simulink model "bd_par_auto2"  (Simulink 4.1.1)
settings: Solver=ode1  SolverMode=SingleTasking  StartTime=0.0  StopTime=max(cyc_mph(:,1))  FixedStep=1  MaxStep=1  RelTol=1e-3  AbsTol=1e-3
undefined symbols (not defined in the file): air_cp, amb_tmp, cs_charge_deplete_bool, cs_charge_trq, cs_electric_decel_spd, cs_electric_launch_spd_hi, cs_electric_launch_spd_lo, cs_hi_soc, cs_lo_soc, cs_min_trq_frac, cs_off_trq_frac, cyc_avg_time, cyc_cargo_mass, cyc_elevation_init, cyc_filter_bool, cyc_grade, cyc_mph, enable_stop, ess_cap_scale, ess_coulombic_eff, ess_init_soc, ess_max_ah_cap, ess_max_volts, ess_min_volts, ess_mod_airflow, ess_mod_cp, ess_mod_init_tmp, ess_module_mass, ess_module_num, ess_on, ess_res_scale_coef, ess_res_scale_fun, ess_set_tmp, ess_th_calc, ess_th_res_off, ess_th_res_on, ess_tmp, ess_voc, ex_calc, fc_ct_trq, fc_emis, fc_inertia, fc_map_spd, fc_max_trq, fc_on, fc_spd_scale, fc_trq_scale, fc_tstat, fd_inertia, fd_loss, fd_ratio, gb_dnshift_load, gb_dnshift_spd, gb_gears_num, gb_inertia, gb_num_init, gb_ratio, gb_shift_delay, gb_spd_scale, gb_trq_scale ... (+56)
libraries: lib_wheel2 x12, lib_accessory2 x3, lib_etc x2, lib_drive_cycle2 x1, lib_interactive x1, lib_drive_cycle x1, lib_exhaust x1, lib_fuel_converter3 x1
(part 13 of 18)

== system bd_par_auto2/gearbox <gb> old/gearbox model & interface/gearbox model/gearbox controller interface ==
  T_gb_out : Inport  Port=1  LatchInput=off
  w_gb_out : Inport  Port=2  LatchInput=off
  eta_gb : Inport  Port=3  LatchInput=off
  enhancedToWorkspace1 : Subsystem  mask(enhancedToWorkspace){generalName=generalName, specificName=gear_ratio, logFlag=logFlag}
      mask prompts: generalName "General Name [char-evaluated]"; specificName "Specific Name [char-literal]"; logFlag "Enable flag (1=on,0=off)"
      mask help: A wrapper for the Simulink "To Workspace" block that allows you to evaluate the name of the variable to log to workspace. This is useful to avoid the double logging errors that occur when you pull in two library models that attempt to log to the same variable.
      mask init:
      | enhancedToWsMaker
      settings: CopyFcn=breakLinkCopyFcn  ParentCloseFcn=breakLinkParCloseFcn  RTWFcnNameOpts=Auto  RTWFileNameOpts=Auto
      mask Help:
      | <h2>Enhanced To Workspace Block</h2>
      | <h3>Parameters</h3>
      | <UL>
      | <li><b>General Name:</b> This is the more general name of the variable. Variables are saved to the workspace as <i>generalName_specificName</i>. Note that this is an evaluated variable. If you would like to type in the value directly, it must be surrounded with single quotes. Otherwise you can input the name of a variable containing a char string.</li>
      | <li><b>Specific Name:</b> This is the specific name of the variable. Note that this is input as a char literal (i.e., you don't need quotes).</li>
      | <li><b>Enable Flag:</b> This flag should have the value of 0 or 1. If 0, the variable will not be logged to the workspace. If 1, the variable will be logged. This is done so that variable logging can be turned off to improve speed.</li>
      | </ul>
      | <h3>Overview</h3>
      | <p>The enhanced to workspace block was put together to allow one to dynamically resolve variable names at run time in simulink. This is most powerful when used in conjunction with a masked subsystem to allow multiple instances of that masked subsytem to be used in the same model. The strategy is to set the generalName in the block mask which will allow the block to change the general name for all variable logging on the fly.
      | <h3>Helper Files</h3>
      | <p>Three m-files are required by the enhancedToWorkspace block. These files are located in the &lt; ADVISOR root &gt;/GUI directory :
      | <ul>
      | <li><i>enhancedToWsMaker.m</i> This file runs the mask initialization for the block</li>
      | <li><i>breakLinkCopyFcn.m</i> This file is used by the block callback when the simulink block is copied. It is necessary to break the link to the enhancedToWorkspace similar to the To Workspace block in order for it to be able to configure itself. (Try copying simulink's To Workspace block--it is impossible to make a link)</li>
      | <li><i>breakLinkParCloseFcn.m</i> This file is similar to the breakLinkCopyFcn and is used when a parent system is closed</li>
      | </ul>
      | <hr>
      | 
      | <p>Created 2003-Jan-21, Michael Patrick O'Keefe, NREL</p>
      mask Display: disp([generalName,'_',specificName])
  enhancedToWorkspace8 : Subsystem  mask(enhancedToWorkspace){generalName=generalName, specificName=shifting, logFlag=logFlag}
      mask prompts: generalName "General Name [char-evaluated]"; specificName "Specific Name [char-literal]"; logFlag "Enable flag (1=on,0=off)"
      mask help: A wrapper for the Simulink "To Workspace" block that allows you to evaluate the name of the variable to log to workspace. This is useful to avoid the double logging errors that occur when you pull in two library models that attempt to log to the same variable.
      mask init:
      | enhancedToWsMaker
      settings: CopyFcn=breakLinkCopyFcn  ParentCloseFcn=breakLinkParCloseFcn  RTWFcnNameOpts=Auto  RTWFileNameOpts=Auto
      mask Help:
      | <h2>Enhanced To Workspace Block</h2>
      | <h3>Parameters</h3>
      | <UL>
      | <li><b>General Name:</b> This is the more general name of the variable. Variables are saved to the workspace as <i>generalName_specificName</i>. Note that this is an evaluated variable. If you would like to type in the value directly, it must be surrounded with single quotes. Otherwise you can input the name of a variable containing a char string.</li>
      | <li><b>Specific Name:</b> This is the specific name of the variable. Note that this is input as a char literal (i.e., you don't need quotes).</li>
      | <li><b>Enable Flag:</b> This flag should have the value of 0 or 1. If 0, the variable will not be logged to the workspace. If 1, the variable will be logged. This is done so that variable logging can be turned off to improve speed.</li>
      | </ul>
      | <h3>Overview</h3>
      | <p>The enhanced to workspace block was put together to allow one to dynamically resolve variable names at run time in simulink. This is most powerful when used in conjunction with a masked subsystem to allow multiple instances of that masked subsytem to be used in the same model. The strategy is to set the generalName in the block mask which will allow the block to change the general name for all variable logging on the fly.
      | <h3>Helper Files</h3>
      | <p>Three m-files are required by the enhancedToWorkspace block. These files are located in the &lt; ADVISOR root &gt;/GUI directory :
      | <ul>
      | <li><i>enhancedToWsMaker.m</i> This file runs the mask initialization for the block</li>
      | <li><i>breakLinkCopyFcn.m</i> This file is used by the block callback when the simulink block is copied. It is necessary to break the link to the enhancedToWorkspace similar to the To Workspace block in order for it to be able to configure itself. (Try copying simulink's To Workspace block--it is impossible to make a link)</li>
      | <li><i>breakLinkParCloseFcn.m</i> This file is similar to the breakLinkCopyFcn and is used when a parent system is closed</li>
      | </ul>
      | <hr>
      | 
      | <p>Created 2003-Jan-21, Michael Patrick O'Keefe, NREL</p>
      mask Display: disp([generalName,'_',specificName])
  gear_ratio : Outport  Port=1  InitialOutput=0
  shifting : Outport  Port=2  InitialOutput=0
  tag scope: T_gb_out=scoped, eta_gb=scoped, w_gb_out=scoped
  wires:
  [shifting] -> enhancedToWorkspace8/1(In1), shifting/1
  T_gb_out/1 -> [T_gb_out]
  w_gb_out/1 -> [w_gb_out]
  eta_gb/1 -> [eta_gb]
  [gear_ratio] -> enhancedToWorkspace1/1(In1), gear_ratio/1

== system bd_par_auto2/gearbox <gb> old/gearbox model & interface/gearbox model/gearing (Nm) (rad/s) ==
  "output shaft torque and speed  (Nm), (rad/s)" : Inport  Port=1  LatchInput=off
  gear ratio : Inport  Port=2  LatchInput=off
  Demux : Demux  Outputs=2  BusSelectionMode=off
  Fcn1 : Fcn  Expr=1/u
  Product2 : Product  Inputs=2  Multiplication=Element-wise(.*)  SaturateOnIntegerOverflow=on
  Product3 : Product  Inputs=2  Multiplication=Element-wise(.*)  SaturateOnIntegerOverflow=on
  input shaft torque (Nm) : Outport  Port=1  InitialOutput=0
  input shaft speed (rad/s) : Outport  Port=2  InitialOutput=0
  wires:
  Demux/2 -> Product3/1
  Demux/1 -> Product2/1
  gear ratio/1 -> Product3/2, Fcn1/1
  "output shaft torque and speed  (Nm), (rad/s)"/1 -> Demux/1
  Fcn1/1 -> Product2/2
  Product2/1 -> input shaft torque (Nm)/1
  Product3/1 -> input shaft speed (rad/s)/1

== system bd_par_auto2/gearbox <gb> old/gearbox model & interface/gearbox model/gearing (Nm) (rad/s)1 ==
  input shaft torque (Nm) : Inport  Port=1  LatchInput=off
  input shaft speed (rad/s) : Inport  Port=2  LatchInput=off
  gear ratio : Inport  Port=3  LatchInput=off
  Fcn1 : Fcn  Expr=1/u
  Product2 : Product  Inputs=2  Multiplication=Element-wise(.*)  SaturateOnIntegerOverflow=on
  Product3 : Product  Inputs=2  Multiplication=Element-wise(.*)  SaturateOnIntegerOverflow=on
  output shaft torque (Nm) : Outport  Port=1  InitialOutput=0
  output shaft speed (rad/s) : Outport  Port=2  InitialOutput=0
  wires:
  input shaft speed (rad/s)/1 -> Product3/2
  input shaft torque (Nm)/1 -> Product2/1
  Product2/1 -> output shaft torque (Nm)/1
  Product3/1 -> output shaft speed (rad/s)/1
  gear ratio/1 -> Fcn1/1, Product2/2
  Fcn1/1 -> Product3/1

== system bd_par_auto2/gearbox <gb> old/gearbox model & interface/gearbox model/help ==

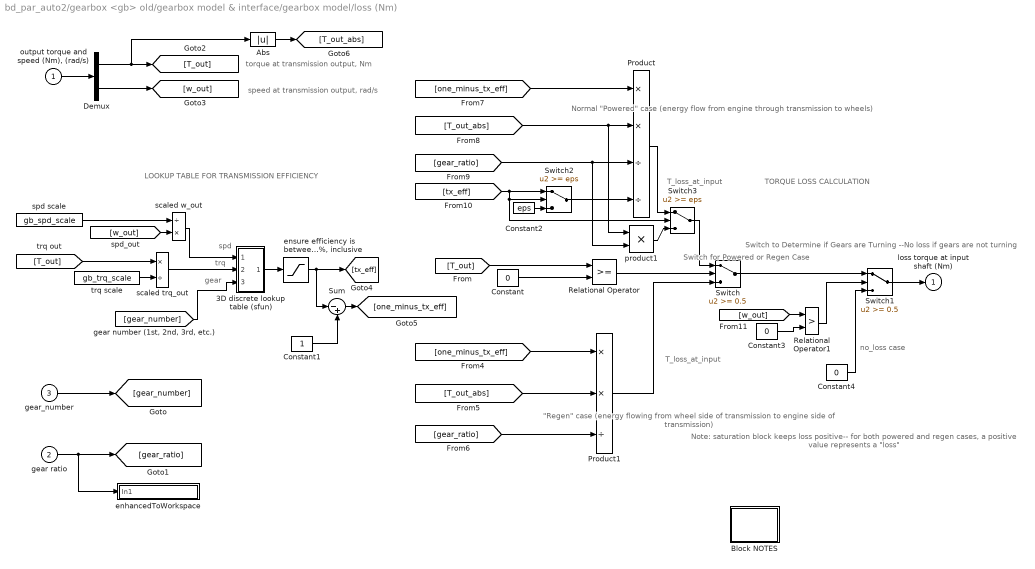
== system bd_par_auto2/gearbox <gb> old/gearbox model & interface/gearbox model/loss (Nm) ==
  note: LOOKUP TABLE FOR TRANSMISSION EFFICIENCY
  note: T_loss_at_input
  note: "Regen" case
      | (energy flowing from
      | wheel side of transmission
      | to engine side of transmission)
  note: T_loss_at_input
  note: Normal "Powered" case
      | (energy flow from engine
      | through transmission to wheels)
  note: Switch to Determine
      | if Gears are Turning
      | --No loss if gears
      | are not turning
  note: Switch for Powered
      |  or Regen Case
  note: Note: saturation block keeps
      | loss positive-- for both powered
      | and regen cases, a
      | positive value represents a "loss"
  note: no_loss case
  note: speed at transmission output, rad/s
  note: torque at transmission output, Nm
  note: spd
  note: trq
  note: gear
  note: TORQUE LOSS CALCULATION
  "output torque and speed (Nm), (rad/s)" : Inport  Port=1  LatchInput=off
  gear ratio : Inport  Port=2  LatchInput=off
  gear_number : Inport  Port=3  LatchInput=off
  3D discrete lookup table (sfun) : Subsystem  mask{tx_map_spd=tx_map_spd, tx_map_trq=tx_map_trq, tx_eff_map=tx_eff_map}
      mask prompts: tx_map_spd "Row Lookup"; tx_map_trq "Column Lookup"; tx_eff_map "Lookup Matrix"
      settings: RTWFcnNameOpts=Auto  RTWFileNameOpts=Auto
  Abs : Abs  SaturateOnIntegerOverflow=on
  Block NOTES : Subsystem
      settings: RTWFcnNameOpts=Auto  RTWFileNameOpts=Auto
      mask Display: disp('Block\nNOTES')
  Constant : Constant  Value=0
  Constant1 : Constant  Value=1
  Constant2 : Constant  Value=eps
  Constant3 : Constant  Value=0
  Constant4 : Constant  Value=0
  Demux : Demux  Outputs=2  BusSelectionMode=off
  Product : Product  Inputs=**//  Multiplication=Element-wise(.*)  SaturateOnIntegerOverflow=on
  Product1 : Product  Inputs=**/  Multiplication=Element-wise(.*)  SaturateOnIntegerOverflow=on
  Relational Operator : RelationalOperator  Operator=>=
  Relational Operator1 : RelationalOperator  Operator=>
  Sum : Sum  Inputs=|-+  SaturateOnIntegerOverflow=on
  Switch : Switch  Threshold=0.5
  Switch1 : Switch  Threshold=0.5
  Switch2 : Switch  Threshold=eps
  Switch3 : Switch  Threshold=eps
  enhancedToWorkspace : Subsystem  TreatAsAtomicUnit=on  mask(enhancedToWorkspace){generalName=generalName, specificName=current_gear_ratio, logFlag=logFlag}
      mask prompts: generalName "General Name [char-evaluated]"; specificName "Specific Name [char-literal]"; logFlag "Enable flag (1=on,0=off)"
      mask help: A wrapper for the Simulink "To Workspace" block that allows you to evaluate the name of the variable to log to workspace. This is useful to avoid the double logging errors that occur when you pull in two library models that attempt to log to the same variable.
      mask init:
      | enhancedToWsMaker
      settings: CopyFcn=breakLinkCopyFcn  ParentCloseFcn=breakLinkParCloseFcn  RTWFcnNameOpts=Auto  RTWFileNameOpts=Auto
      mask Help:
      | <h2>Enhanced To Workspace Block</h2>
      | <h3>Parameters</h3>
      | <UL>
      | <li><b>General Name:</b> This is the more general name of the variable. Variables are saved to the workspace as <i>generalName_specificName</i>. Note that this is an evaluated variable. If you would like to type in the value directly, it must be surrounded with single quotes. Otherwise you can input the name of a variable containing a char string.</li>
      | <li><b>Specific Name:</b> This is the specific name of the variable. Note that this is input as a char literal (i.e., you don't need quotes).</li>
      | <li><b>Enable Flag:</b> This flag should have the value of 0 or 1. If 0, the variable will not be logged to the workspace. If 1, the variable will be logged. This is done so that variable logging can be turned off to improve speed.</li>
      | </ul>
      | <h3>Overview</h3>
      | <p>The enhanced to workspace block was put together to allow one to dynamically resolve variable names at run time in simulink. This is most powerful when used in conjunction with a masked subsystem to allow multiple instances of that masked subsytem to be used in the same model. The strategy is to set the generalName in the block mask which will allow the block to change the general name for all variable logging on the fly.
      | <h3>Helper Files</h3>
      | <p>Three m-files are required by the enhancedToWorkspace block. These files are located in the &lt; ADVISOR root &gt;/GUI directory :
      | <ul>
      | <li><i>enhancedToWsMaker.m</i> This file runs the mask initialization for the block</li>
      | <li><i>breakLinkCopyFcn.m</i> This file is used by the block callback when the simulink block is copied. It is necessary to break the link to the enhancedToWorkspace similar to the To Workspace block in order for it to be able to configure itself. (Try copying simulink's To Workspace block--it is impossible to make a link)</li>
      | <li><i>breakLinkParCloseFcn.m</i> This file is similar to the breakLinkCopyFcn and is used when a parent system is closed</li>
      | </ul>
      | <hr>
      | 
      | <p>Created 2003-Jan-21, Michael Patrick O'Keefe, NREL</p>
      | 
      | <!--
      | <VARDEF>
      | <H3>var_name</H3>
      | <UL>
      | <LI><B>data type</B> data type here</LI>
      | <LI><B>units</B> units here</LI>
      | <LI><B>vehicle type</B> vehicle type here</LI>
      | <LI><B>description</B> description here</LI>
      | </UL>
      | </VARDEF>
      | -->
      mask Display: disp([generalName,'_',specificName])
  "ensure efficiency is between  0% and 100%, inclusive" : Saturate  UpperLimit=1  LowerLimit=0  LinearizeAsGain=on
  product1 : Product  Inputs=2  Multiplication=Element-wise(.*)  SaturateOnIntegerOverflow=on
  scaled trq_out : Product  Inputs=*/  Multiplication=Element-wise(.*)  SaturateOnIntegerOverflow=on
  scaled w_out : Product  Inputs=/*  Multiplication=Element-wise(.*)  SaturateOnIntegerOverflow=on
  spd scale : Constant  Value=gb_spd_scale
  trq scale : Constant  Value=gb_trq_scale
  loss torque at input shaft (Nm) : Outport  Port=1  InitialOutput=0
  wires:
  "output torque and speed (Nm), (rad/s)"/1 -> Demux/1
  Demux/2 -> [w_out]
  [gear_number] -> 3D discrete lookup table (sfun)/3("gear_number  (e.g., 1, 2, 3)")
  Relational Operator/1 -> Switch/2
  Constant/1 -> Relational Operator/2
  [T_out] -> Relational Operator/1
  Product1/1 -> Switch/3
  [one_minus_tx_eff] -> Product1/1
  [gear_ratio] -> Product1/3
  [T_out_abs] -> Product1/2
  [one_minus_tx_eff] -> Product/1
  [T_out_abs] -> Product/2, product1/1
  [gear_ratio] -> Product/3, product1/2
  Switch1/1 -> loss torque at input shaft (Nm)/1
  Constant4/1 -> Switch1/3
  [w_out] -> Relational Operator1/1
  Constant3/1 -> Relational Operator1/2
  Relational Operator1/1 -> Switch1/2
  Demux/1 -> [T_out], Abs/1
  Abs/1 -> [T_out_abs]
  Switch/1 -> Switch1/1
  3D discrete lookup table (sfun)/1(tx_eff) -> "ensure efficiency is between  0% and 100%, inclusive"/1
  "ensure efficiency is between  0% and 100%, inclusive"/1 -> [tx_eff], Sum/1
  scaled w_out/1 -> 3D discrete lookup table (sfun)/1(lookup speed (rad/s))
  [T_out] -> scaled trq_out/1
  scaled trq_out/1 -> 3D discrete lookup table (sfun)/2(lookup trq (Nm))
  trq scale/1 -> scaled trq_out/2
  Constant1/1 -> Sum/2
  Sum/1 -> [one_minus_tx_eff]
  [w_out] -> scaled w_out/2
  spd scale/1 -> scaled w_out/1
  gear ratio/1 -> enhancedToWorkspace/1(In1), [gear_ratio]
  gear_number/1 -> [gear_number]
  Switch2/1 -> Product/4
  [tx_eff] -> Switch2/1, Switch2/2, Switch3/2
  Constant2/1 -> Switch2/3
  Switch3/1 -> Switch/1
  Product/1 -> Switch3/1
  product1/1 -> Switch3/3

== system bd_par_auto2/hydraulic torque converter <htc> HEV/HTC for parallel HEV and Interface/model for parallel HEV/Block NOTES ==
  note: This block predicts the relative speed of the HTC input (pump) and output
      | (turbine).  Torque converter lockup is modeled.

== system bd_par_auto2/hydraulic torque converter <htc> HEV/HTC for parallel HEV and Interface/model for parallel HEV/SR ==
  T,w req out : Inport  Port=1  LatchInput=off
  w in : Inport  Port=2  LatchInput=off
  >0 : Saturate  UpperLimit=inf  LowerLimit=eps  LinearizeAsGain=on
  Constant : Constant  Orientation=left  Value=0
  Constant1 : Constant  Value=vc_idle_spd+eps
  Constant3 : Constant  Value=1
  K_adv : Subsystem
      settings: RTWFcnNameOpts=Auto  RTWFileNameOpts=Auto
  K_adv_coast : Subsystem
      settings: RTWFcnNameOpts=Auto  RTWFileNameOpts=Auto
  Logical Operator : Logic  Operator=NOT  Inputs=1
  Logical Operator1 : Logic  Operator=NOT  Inputs=1
  MinMax : MinMax  Function=min  Inputs=2
  Relational Operator : RelationalOperator  Operator=>=
  SR Look-Up Table SR=wout/win : Lookup  InputValues=htc_k_adv  OutputValues=htc_sr
  SR Look-Up Table SR=wout/win coast : Lookup  InputValues=fliplr(htc_k_adv_coast)  OutputValues=fliplr(htc_sr_coast)
  SRmax= wout/win,min : Product  Inputs=*/  Multiplication=Element-wise(.*)  SaturateOnIntegerOverflow=on
  T : Selector  InputType=Vector  ElementSrc=Internal  Elements=1  RowSrc=Internal  Rows=1  ColumnSrc=Internal  Columns=1  InputPortWidth=2
  enhancedToWorkspace : Subsystem  TreatAsAtomicUnit=on  mask(enhancedToWorkspace){generalName=generalName, specificName=locked, logFlag=logFlag}
      mask prompts: generalName "General Name [char-evaluated]"; specificName "Specific Name [char-literal]"; logFlag "Enable flag (1=on,0=off)"
      mask help: A wrapper for the Simulink "To Workspace" block that allows you to evaluate the name of the variable to log to workspace. This is useful to avoid the double logging errors that occur when you pull in two library models that attempt to log to the same variable.
      mask init:
      | enhancedToWsMaker
      settings: CopyFcn=breakLinkCopyFcn  ParentCloseFcn=breakLinkParCloseFcn  RTWFcnNameOpts=Auto  RTWFileNameOpts=Auto
      mask Help:
      | <h2>Enhanced To Workspace Block</h2>
      | <h3>Parameters</h3>
      | <UL>
      | <li><b>General Name:</b> This is the more general name of the variable. Variables are saved to the workspace as <i>generalName_specificName</i>. Note that this is an evaluated variable. If you would like to type in the value directly, it must be surrounded with single quotes. Otherwise you can input the name of a variable containing a char string.</li>
      | <li><b>Specific Name:</b> This is the specific name of the variable. Note that this is input as a char literal (i.e., you don't need quotes).</li>
      | <li><b>Enable Flag:</b> This flag should have the value of 0 or 1. If 0, the variable will not be logged to the workspace. If 1, the variable will be logged. This is done so that variable logging can be turned off to improve speed.</li>
      | </ul>
      | <h3>Overview</h3>
      | <p>The enhanced to workspace block was put together to allow one to dynamically resolve variable names at run time in simulink. This is most powerful when used in conjunction with a masked subsystem to allow multiple instances of that masked subsytem to be used in the same model. The strategy is to set the generalName in the block mask which will allow the block to change the general name for all variable logging on the fly.
      | <h3>Helper Files</h3>
      | <p>Three m-files are required by the enhancedToWorkspace block. These files are located in the &lt; ADVISOR root &gt;/GUI directory :
      | <ul>
      | <li><i>enhancedToWsMaker.m</i> This file runs the mask initialization for the block</li>
      | <li><i>breakLinkCopyFcn.m</i> This file is used by the block callback when the simulink block is copied. It is necessary to break the link to the enhancedToWorkspace similar to the To Workspace block in order for it to be able to configure itself. (Try copying simulink's To Workspace block--it is impossible to make a link)</li>
      | <li><i>breakLinkParCloseFcn.m</i> This file is similar to the breakLinkCopyFcn and is used when a parent system is closed</li>
      | </ul>
      | <hr>
      | 
      | <p>Created 2003-Jan-21, Michael Patrick O'Keefe, NREL</p>
      | 
      | <!--
      | <VARDEF>
      | <H3>var_name</H3>
      | <UL>
      | <LI><B>data type</B> data type here</LI>
      | <LI><B>units</B> units here</LI>
      | <LI><B>vehicle type</B> vehicle type here</LI>
      | <LI><B>description</B> description here</LI>
      | </UL>
      | </VARDEF>
      | -->
      mask Display: disp([generalName,'_',specificName])
  enhancedToWorkspace1 : Subsystem  TreatAsAtomicUnit=on  mask(enhancedToWorkspace){generalName=generalName, specificName=coasting, logFlag=logFlag}
      mask prompts: generalName "General Name [char-evaluated]"; specificName "Specific Name [char-literal]"; logFlag "Enable flag (1=on,0=off)"
      mask help: A wrapper for the Simulink "To Workspace" block that allows you to evaluate the name of the variable to log to workspace. This is useful to avoid the double logging errors that occur when you pull in two library models that attempt to log to the same variable.
      mask init:
      | enhancedToWsMaker
      settings: CopyFcn=breakLinkCopyFcn  ParentCloseFcn=breakLinkParCloseFcn  RTWFcnNameOpts=Auto  RTWFileNameOpts=Auto
      mask Help:
      | <h2>Enhanced To Workspace Block</h2>
      | <h3>Parameters</h3>
      | <UL>
      | <li><b>General Name:</b> This is the more general name of the variable. Variables are saved to the workspace as <i>generalName_specificName</i>. Note that this is an evaluated variable. If you would like to type in the value directly, it must be surrounded with single quotes. Otherwise you can input the name of a variable containing a char string.</li>
      | <li><b>Specific Name:</b> This is the specific name of the variable. Note that this is input as a char literal (i.e., you don't need quotes).</li>
      | <li><b>Enable Flag:</b> This flag should have the value of 0 or 1. If 0, the variable will not be logged to the workspace. If 1, the variable will be logged. This is done so that variable logging can be turned off to improve speed.</li>
      | </ul>
      | <h3>Overview</h3>
      | <p>The enhanced to workspace block was put together to allow one to dynamically resolve variable names at run time in simulink. This is most powerful when used in conjunction with a masked subsystem to allow multiple instances of that masked subsytem to be used in the same model. The strategy is to set the generalName in the block mask which will allow the block to change the general name for all variable logging on the fly.
      | <h3>Helper Files</h3>
      | <p>Three m-files are required by the enhancedToWorkspace block. These files are located in the &lt; ADVISOR root &gt;/GUI directory :
      | <ul>
      | <li><i>enhancedToWsMaker.m</i> This file runs the mask initialization for the block</li>
      | <li><i>breakLinkCopyFcn.m</i> This file is used by the block callback when the simulink block is copied. It is necessary to break the link to the enhancedToWorkspace similar to the To Workspace block in order for it to be able to configure itself. (Try copying simulink's To Workspace block--it is impossible to make a link)</li>
      | <li><i>breakLinkParCloseFcn.m</i> This file is similar to the breakLinkCopyFcn and is used when a parent system is closed</li>
      | </ul>
      | <hr>
      | 
      | <p>Created 2003-Jan-21, Michael Patrick O'Keefe, NREL</p>
      | 
      | <!--
      | <VARDEF>
      | <H3>var_name</H3>
      | <UL>
      | <LI><B>data type</B> data type here</LI>
      | <LI><B>units</B> units here</LI>
      | <LI><B>vehicle type</B> vehicle type here</LI>
      | <LI><B>description</B> description here</LI>
      | </UL>
      | </VARDEF>
      | -->
      mask Display: disp([generalName,'_',specificName])
  if coasting : Switch  Threshold=eps
  "locked up, then SR=1" : Switch  Threshold=eps
  min,max : Saturate  UpperLimit=inf  LowerLimit=1  LinearizeAsGain=on
  shifting SR : Subsystem
      settings: RTWFcnNameOpts=Auto  RTWFileNameOpts=Auto
  wout,req : Selector  InputType=Vector  ElementSrc=Internal  Elements=2  RowSrc=Internal  Rows=1  ColumnSrc=Internal  Columns=1  InputPortWidth=2
  SR : Outport  Port=1  InitialOutput=0
  coasting : Outport  Port=2  InitialOutput=0
  wires:
  Relational Operator/1 -> if coasting/2, Logical Operator1/1
  [locked_up] -> enhancedToWorkspace/1(In1), Logical Operator/1
  T,w req out/1 -> T/1, K_adv_coast/1("Req'd output trq and spd (Nm), (rad/s)"), wout,req/1, K_adv/1("Req'd output trq and spd (Nm), (rad/s)"), shifting SR/1(T,w req out)
  SR Look-Up Table SR=wout/win coast/1 -> min,max/1
  Constant/1 -> Relational Operator/2
  T/1 -> Relational Operator/1
  Logical Operator/1 -> "locked up, then SR=1"/2
  Constant3/1 -> "locked up, then SR=1"/3
  SR Look-Up Table SR=wout/win/1 -> "locked up, then SR=1"/1
  w in/1 -> shifting SR/2(w in)
  "locked up, then SR=1"/1 -> shifting SR/3(SR)
  shifting SR/1(SR limited) -> if coasting/1
  SRmax= wout/win,min/1 -> MinMax/2
  Constant1/1 -> SRmax= wout/win,min/2
  wout,req/1 -> SRmax= wout/win,min/1
  min,max/1 -> MinMax/1
  MinMax/1 -> if coasting/3
  K_adv_coast/1(K_adv_coast) -> SR Look-Up Table SR=wout/win coast/1
  if coasting/1 -> >0/1
  >0/1 -> SR/1
  Logical Operator1/1 -> enhancedToWorkspace1/1(In1), coasting/1
  K_adv/1(K_adv) -> SR Look-Up Table SR=wout/win/1

== system bd_par_auto2/hydraulic torque converter <htc> HEV/HTC for parallel HEV and Interface/model for parallel HEV/T, shifting ==
  TR : Inport  Port=1  LatchInput=off
  Req'd  input trq : Inport  Port=2  LatchInput=off
  Req'd output trq : Inport  Port=3  LatchInput=off
  htc_spd_in_a : Inport  Port=4  LatchInput=off
  SR : Inport  Port=5  LatchInput=off
  Memory : Memory  X0=0  InheritSampleTime=off
      settings: RTWStateStorageClass=Auto
  Memory1 : Memory  X0=0  InheritSampleTime=off
      settings: RTWStateStorageClass=Auto
  MinMax : MinMax  Function=min  Inputs=2
  TR Look-Up Table TR=Tout/Tin : Lookup  InputValues=htc_sr  OutputValues=htc_tr
  T_max : Subsystem
      settings: RTWFcnNameOpts=Auto  RTWFileNameOpts=Auto
  Tin*TR= Tout,req : Product  Inputs=2  Multiplication=Element-wise(.*)  SaturateOnIntegerOverflow=on
  engine speed estimator : Subsystem
      settings: RTWFcnNameOpts=Auto  RTWFileNameOpts=Auto
  "shifting, override zero Trequest" : Switch  Threshold=eps
  T req : Outport  Port=1
  wires:
  [shifting] -> "shifting, override zero Trequest"/2
  Req'd output trq/1 -> "shifting, override zero Trequest"/3
  htc_spd_in_a/1 -> engine speed estimator/1(htc_spd_in_a)
  SR/1 -> Memory1/1
  Memory1/1 -> TR Look-Up Table TR=Tout/Tin/1
  engine speed estimator/1(Out1) -> T_max/1(w_APU)
  MinMax/1 -> T req/1
  TR Look-Up Table TR=Tout/Tin/1 -> T_max/2(TR)
  "shifting, override zero Trequest"/1 -> MinMax/1
  T_max/1(T_max max gain from htc) -> MinMax/2
  Memory/1 -> "shifting, override zero Trequest"/1
  Req'd  input trq/1 -> Tin*TR= Tout,req/1
  TR/1 -> Tin*TR= Tout,req/2
  Tin*TR= Tout,req/1 -> Memory/1

== system bd_par_auto2/hydraulic torque converter <htc> HEV/HTC for parallel HEV and Interface/model for parallel HEV/TR ==
  SR : Inport  Port=1  LatchInput=off
  coasting : Inport  Port=2  LatchInput=off
  1/SR*TR  for coast : Fcn  Expr=1/u
  Constant3 : Constant  Value=1
  Logical Operator : Logic  Operator=NOT  Inputs=1
  Logical Operator1 : Logic  Operator=NOT  Inputs=1
  TR Look-Up Table TR=Tout/Tin : Lookup  InputValues=htc_sr  OutputValues=htc_tr
  TR Look-Up Table TR=Tout/Tin coast : Lookup  InputValues=htc_sr_coast  OutputValues=htc_tr_coast
  To Workspace11 : ToWorkspace  VariableName=htc_efficiency  SampleTime=-1  SaveFormat=Array
  effic=SR*TR : Product  Inputs=**  Multiplication=Element-wise(.*)  SaturateOnIntegerOverflow=on
  if coasting : Switch  Threshold=eps
  if coasting1 : Switch  Threshold=eps
  "locked up, then TR=1" : Switch  Threshold=eps
  min,max : Saturate  UpperLimit=htc_max_coast_tr  LowerLimit=htc_min_coast_tr  LinearizeAsGain=on
  TR : Outport  Port=1  InitialOutput=0
  wires:
  TR Look-Up Table TR=Tout/Tin/1 -> "locked up, then TR=1"/1
  Constant3/1 -> "locked up, then TR=1"/3
  [locked_up] -> Logical Operator/1
  Logical Operator/1 -> "locked up, then TR=1"/2
  "locked up, then TR=1"/1 -> if coasting/1
  TR Look-Up Table TR=Tout/Tin coast/1 -> min,max/1
  min,max/1 -> if coasting/3
  SR/1 -> TR Look-Up Table TR=Tout/Tin coast/1, TR Look-Up Table TR=Tout/Tin/1, effic=SR*TR/1
  coasting/1 -> Logical Operator1/1
  if coasting/1 -> TR/1, effic=SR*TR/2
  Logical Operator1/1 -> if coasting/2, if coasting1/2
  effic=SR*TR/1 -> if coasting1/1, 1/SR*TR  for coast/1
  1/SR*TR  for coast/1 -> if coasting1/3
  if coasting1/1 -> To Workspace11/1

== system bd_par_auto2/hydraulic torque converter <htc> HEV/HTC for parallel HEV and Interface/model for parallel HEV/effect of inertia (Nm) ==
  note: This block computes the torque required to overcome the inertia of the
      | turbine (plus 1/2 fluid in htc).
  turbine/output speed (rad/s) : Inport  Port=1  LatchInput=off
  Constant : Constant  Value=htc_inertia
  Product : Product  Inputs=2  Multiplication=Element-wise(.*)  SaturateOnIntegerOverflow=on
  d/dt : Derivative
  inertia torque (Nm) : Outport  Port=1  InitialOutput=0
  wires:
  d/dt/1 -> Product/1
  turbine/output speed (rad/s)/1 -> d/dt/1
  Constant/1 -> Product/2
  Product/1 -> inertia torque (Nm)/1

== system bd_par_auto2/hydraulic torque converter <htc> HEV/HTC for parallel HEV and Interface/model for parallel HEV/enhancedToWorkspace ==
  In1 : Inport  Port=1  LatchInput=off
  To Workspace : ToWorkspace  VariableName=htc_spd_in_a  SampleTime=-1  SaveFormat=Array
  wires:
  In1/1 -> To Workspace/1

== system bd_par_auto2/hydraulic torque converter <htc> HEV/HTC for parallel HEV and Interface/model for parallel HEV/enhancedToWorkspace1 ==
  In1 : Inport  Port=1  LatchInput=off
  To Workspace : ToWorkspace  VariableName=htc_trq_in_a  SampleTime=-1  SaveFormat=Array
  wires:
  In1/1 -> To Workspace/1

== system bd_par_auto2/hydraulic torque converter <htc> HEV/HTC for parallel HEV and Interface/model for parallel HEV/enhancedToWorkspace10 ==
  In1 : Inport  Port=1  LatchInput=off
  To Workspace : ToWorkspace  VariableName=htc_trq_in_r  SampleTime=-1  SaveFormat=Array
  wires:
  In1/1 -> To Workspace/1

== system bd_par_auto2/hydraulic torque converter <htc> HEV/HTC for parallel HEV and Interface/model for parallel HEV/enhancedToWorkspace2 ==
  In1 : Inport  Port=1  LatchInput=off
  To Workspace : ToWorkspace  VariableName=htc_sr_hist  SampleTime=-1  SaveFormat=Array
  wires:
  In1/1 -> To Workspace/1

== system bd_par_auto2/hydraulic torque converter <htc> HEV/HTC for parallel HEV and Interface/model for parallel HEV/enhancedToWorkspace3 ==
  In1 : Inport  Port=1  LatchInput=off
  To Workspace : ToWorkspace  VariableName=htc_tr_hist  SampleTime=-1  SaveFormat=Array
  wires:
  In1/1 -> To Workspace/1

== system bd_par_auto2/hydraulic torque converter <htc> HEV/HTC for parallel HEV and Interface/model for parallel HEV/enhancedToWorkspace4 ==
  In1 : Inport  Port=1  LatchInput=off
  To Workspace : ToWorkspace  VariableName=htc_trq_inertia  SampleTime=-1  SaveFormat=Array
  wires:
  In1/1 -> To Workspace/1

== system bd_par_auto2/hydraulic torque converter <htc> HEV/HTC for parallel HEV and Interface/model for parallel HEV/enhancedToWorkspace5 ==
  In1 : Inport  Port=1  LatchInput=off
  To Workspace : ToWorkspace  VariableName=htc_trq_out_a  SampleTime=-1  SaveFormat=Array
  wires:
  In1/1 -> To Workspace/1

== system bd_par_auto2/hydraulic torque converter <htc> HEV/HTC for parallel HEV and Interface/model for parallel HEV/enhancedToWorkspace6 ==
  In1 : Inport  Port=1  LatchInput=off
  To Workspace : ToWorkspace  VariableName=htc_spd_out_a  SampleTime=-1  SaveFormat=Array
  wires:
  In1/1 -> To Workspace/1

== system bd_par_auto2/hydraulic torque converter <htc> HEV/HTC for parallel HEV and Interface/model for parallel HEV/enhancedToWorkspace7 ==
  In1 : Inport  Port=1  LatchInput=off
  To Workspace : ToWorkspace  VariableName=htc_trq_out_r  SampleTime=-1  SaveFormat=Array
  wires:
  In1/1 -> To Workspace/1

== system bd_par_auto2/hydraulic torque converter <htc> HEV/HTC for parallel HEV and Interface/model for parallel HEV/enhancedToWorkspace8 ==
  In1 : Inport  Port=1  LatchInput=off
  To Workspace : ToWorkspace  VariableName=htc_spd_out_r  SampleTime=-1  SaveFormat=Array
  wires:
  In1/1 -> To Workspace/1

== system bd_par_auto2/hydraulic torque converter <htc> HEV/HTC for parallel HEV and Interface/model for parallel HEV/enhancedToWorkspace9 ==
  In1 : Inport  Port=1  LatchInput=off
  To Workspace : ToWorkspace  VariableName=htc_spd_in_r  SampleTime=-1  SaveFormat=Array
  wires:
  In1/1 -> To Workspace/1

== system bd_par_auto2/motor/controller <mc>/motor model & interface/mc model/Block NOTES ==
  note: Available torque is computed from available power by assuming that the ratio of rotor torque to input
      | (electric) power is the same for the actual/achievable situation as was computed for the request.  This
      | is mathematically equivalent to assuming that the motor/controller efficiency.  Rotor speed for the
      | actual/achievable calculations is as computed in the 'request' branch.
  note: This motor/controller model includes loss data, rotational inertia, and performance limits.

== system bd_par_auto2/motor/controller <mc>/motor model & interface/mc model/N-m drive torque per W input ==
  req'd input power (W) : Inport  Port=1  LatchInput=off
  req'd rotor drive torque (Nm) : Inport  Port=2  LatchInput=off
  Block NOTES : Subsystem
      settings: RTWFcnNameOpts=Auto  RTWFileNameOpts=Auto
      mask Display: disp('Block\nNOTES')
  Constant : Constant  Value=eps
  Constant1 : Constant  Value=0
  Constant2 : Constant  Value=inf
  Product : Product  Inputs=/*  Multiplication=Element-wise(.*)  SaturateOnIntegerOverflow=on
  Relational Operator : RelationalOperator  Operator=~=
  Sum : Sum  Inputs=++  SaturateOnIntegerOverflow=on
  Switch : Switch  Threshold=eps
  Nm per W : Outport  Port=1  InitialOutput=0
  wires:
  Constant2/1 -> Switch/3
  Constant1/1 -> Relational Operator/2
  req'd input power (W)/1 -> Relational Operator/1, Sum/2
  Sum/1 -> Product/1
  Switch/1 -> Nm per W/1
  Relational Operator/1 -> Switch/2
  Product/1 -> Switch/1
  req'd rotor drive torque (Nm)/1 -> Product/2
  Constant/1 -> Sum/1

== system bd_par_auto2/motor/controller <mc>/motor model & interface/mc model/documentation10 ==

== system bd_par_auto2/motor/controller <mc>/motor model & interface/mc model/effect of inertia (Nm) ==
  mc_spd_out_a : Inport  Port=1  LatchInput=off
  Block NOTES : Subsystem
      settings: RTWFcnNameOpts=Auto  RTWFileNameOpts=Auto
      mask Display: disp('Block\nNOTES')
  Constant : Constant  Value=eps
  Constant1 : Constant  Value=max(mc_max_trq)*mc_trq_scale*mc_overtrq_factor
  Constant2 : Constant  Orientation=left  Value=gb_ratio(1)*fd_ratio/wh_radius
  Gain : Gain  Gain=mc_inertia  Multiplication=Element-wise(K.*u)  SaturateOnIntegerOverflow=on
  Memory : Memory  X0=0  InheritSampleTime=off
      settings: RTWStateStorageClass=Auto
  MinMax : MinMax  Function=min  Inputs=2
  Product : Product  Inputs=2  Multiplication=Element-wise(.*)  SaturateOnIntegerOverflow=on
  Sum : Sum  Inputs=++  SaturateOnIntegerOverflow=on
  Switch : Switch  Threshold=eps
  alpha : Derivative
  motor inertia as a function of total vehicle inertia (generous approximation) : Subsystem  Orientation=up
      settings: RTWFcnNameOpts=Auto  RTWFileNameOpts=Auto
  overall gear ratio / wh_radius : Product  Inputs=*/  Multiplication=Element-wise(.*)  SaturateOnIntegerOverflow=on
  out_1 : Outport  Port=1  InitialOutput=0
  wires:
  Switch/1 -> overall gear ratio / wh_radius/2
  Constant2/1 -> Switch/3
  [veh_spd_a_rec_prev] -> Switch/2, Sum/1
  Sum/1 -> Switch/1
  Constant/1 -> Sum/2
  motor inertia as a function of total vehicle inertia (generous approximation)/1(Out1) -> Product/2
  Constant1/1 -> Product/1
  overall gear ratio / wh_radius/1 -> motor inertia as a function of total vehicle inertia (generous approximation)/1(gear ratio)
  Product/1 -> MinMax/2
  Gain/1 -> MinMax/1
  MinMax/1 -> out_1/1
  mc_spd_out_a/1 -> alpha/1, Memory/1
  alpha/1 -> Gain/1
  Memory/1 -> overall gear ratio / wh_radius/1

== system bd_par_auto2/motor/controller <mc>/motor model & interface/mc model/enforce torque limit ==
  req'd motor torque (Nm) : Inport  Port=1  LatchInput=off
  limited motor speed (rad/s) : Inport  Port=2  LatchInput=off
  Block NOTES : Subsystem
      settings: RTWFcnNameOpts=Auto  RTWFileNameOpts=Auto
      mask Display: disp('Block\nNOTES')
  MinMax : MinMax  Function=min  Inputs=2
  MinMax1 : MinMax  Function=max  Inputs=2
  Relational Operator2 : RelationalOperator  Operator=~=
  Switch : Switch  Threshold=0
  enhancedToWorkspace : Subsystem  mask(enhancedToWorkspace){generalName=generalName, specificName=max_trq_vec, logFlag=logFlag}
      mask prompts: generalName "General Name [char-evaluated]"; specificName "Specific Name [char-literal]"; logFlag "Enable flag (1=on,0=off)"
      mask help: A wrapper for the Simulink "To Workspace" block that allows you to evaluate the name of the variable to log to workspace. This is useful to avoid the double logging errors that occur when you pull in two library models that attempt to log to the same variable.
      mask init:
      | enhancedToWsMaker
      settings: CopyFcn=breakLinkCopyFcn  ParentCloseFcn=breakLinkParCloseFcn  RTWFcnNameOpts=Auto  RTWFileNameOpts=Auto
      mask Help:
      | <h2>Enhanced To Workspace Block</h2>
      | <h3>Parameters</h3>
      | <UL>
      | <li><b>General Name:</b> This is the more general name of the variable. Variables are saved to the workspace as <i>generalName_specificName</i>. Note that this is an evaluated variable. If you would like to type in the value directly, it must be surrounded with single quotes. Otherwise you can input the name of a variable containing a char string.</li>
      | <li><b>Specific Name:</b> This is the specific name of the variable. Note that this is input as a char literal (i.e., you don't need quotes).</li>
      | <li><b>Enable Flag:</b> This flag should have the value of 0 or 1. If 0, the variable will not be logged to the workspace. If 1, the variable will be logged. This is done so that variable logging can be turned off to improve speed.</li>
      | </ul>
      | <h3>Overview</h3>
      | <p>The enhanced to workspace block was put together to allow one to dynamically resolve variable names at run time in simulink. This is most powerful when used in conjunction with a masked subsystem to allow multiple instances of that masked subsytem to be used in the same model. The strategy is to set the generalName in the block mask which will allow the block to change the general name for all variable logging on the fly.
      | <h3>Helper Files</h3>
      | <p>Three m-files are required by the enhancedToWorkspace block. These files are located in the &lt; ADVISOR root &gt;/GUI directory :
      | <ul>
      | <li><i>enhancedToWsMaker.m</i> This file runs the mask initialization for the block</li>
      | <li><i>breakLinkCopyFcn.m</i> This file is used by the block callback when the simulink block is copied. It is necessary to break the link to the enhancedToWorkspace similar to the To Workspace block in order for it to be able to configure itself. (Try copying simulink's To Workspace block--it is impossible to make a link)</li>
      | <li><i>breakLinkParCloseFcn.m</i> This file is similar to the breakLinkCopyFcn and is used when a parent system is closed</li>
      | </ul>
      | <hr>
      | 
      | <p>Created 2003-Jan-21, Michael Patrick O'Keefe, NREL</p>
      mask Display: disp([generalName,'_',specificName])
  max gen torque : Lookup  InputValues=mc_map_spd*mc_spd_scale  OutputValues=mc_max_gen_trq*mc_overtrq_factor*mc_trq_scale
  max torque : Lookup  InputValues=mc_map_spd*mc_spd_scale  OutputValues=mc_max_trq*mc_overtrq_factor*mc_trq_scale
  limited motor torque (Nm) : Outport  Port=1
  tag scope: mc_trq_limited=scoped
  wires:
  max gen torque/1 -> MinMax1/2
  limited motor speed (rad/s)/1 -> max gen torque/1, max torque/1
  Relational Operator2/1 -> [mc_trq_limited]
  MinMax/1 -> Switch/1
  MinMax1/1 -> Switch/3
  Switch/1 -> limited motor torque (Nm)/1, Relational Operator2/2
  req'd motor torque (Nm)/1 -> MinMax/1, MinMax1/1, Switch/2, Relational Operator2/1
  max torque/1 -> enhancedToWorkspace/1(In1), MinMax/2

== system bd_par_auto2/motor/controller <mc>/motor model & interface/mc model/enhancedToWorkspace ==
  In1 : Inport  Port=1  LatchInput=off
  To Workspace : ToWorkspace  VariableName=mc_pwr_in_a  SampleTime=-1  SaveFormat=Array
  wires:
  In1/1 -> To Workspace/1

== system bd_par_auto2/motor/controller <mc>/motor model & interface/mc model/enhancedToWorkspace1 ==
  In1 : Inport  Port=1  LatchInput=off
  To Workspace : ToWorkspace  VariableName=mc_ni_trq_out_a  SampleTime=-1  SaveFormat=Array
  wires:
  In1/1 -> To Workspace/1

== system bd_par_auto2/motor/controller <mc>/motor model & interface/mc model/enhancedToWorkspace2 ==
  In1 : Inport  Port=1  LatchInput=off
  To Workspace : ToWorkspace  VariableName=mc_spd_out_r  SampleTime=-1  SaveFormat=Array
  wires:
  In1/1 -> To Workspace/1

== system bd_par_auto2/motor/controller <mc>/motor model & interface/mc model/enhancedToWorkspace3 ==
  In1 : Inport  Port=1  LatchInput=off
  To Workspace : ToWorkspace  VariableName=mc_trq_out_r  SampleTime=-1  SaveFormat=Array
  wires:
  In1/1 -> To Workspace/1

== system bd_par_auto2/motor/controller <mc>/motor model & interface/mc model/enhancedToWorkspace4 ==
  In1 : Inport  Port=1  LatchInput=off
  To Workspace : ToWorkspace  VariableName=mc_pwr_loss  SampleTime=-1  SaveFormat=Array
  wires:
  In1/1 -> To Workspace/1

== system bd_par_auto2/motor/controller <mc>/motor model & interface/mc model/enhancedToWorkspace5 ==
  In1 : Inport  Port=1  LatchInput=off
  To Workspace : ToWorkspace  VariableName=mc_mc_tmp  SampleTime=-1  SaveFormat=Array
  wires:
  In1/1 -> To Workspace/1

== system bd_par_auto2/motor/controller <mc>/motor model & interface/mc model/enhancedToWorkspace6 ==
  In1 : Inport  Port=1  LatchInput=off
  To Workspace : ToWorkspace  VariableName=mc_clt_th_pwr  SampleTime=-1  SaveFormat=Array
  wires:
  In1/1 -> To Workspace/1

== system bd_par_auto2/motor/controller <mc>/motor model & interface/mc model/enhancedToWorkspace7 ==
  In1 : Inport  Port=1  LatchInput=off
  To Workspace : ToWorkspace  VariableName=mc_pwr_in_r  SampleTime=-1  SaveFormat=Array
  wires:
  In1/1 -> To Workspace/1

== system bd_par_auto2/motor/controller <mc>/motor model & interface/mc model/enhancedToWorkspace8 ==
  In1 : Inport  Port=1  LatchInput=off
  To Workspace : ToWorkspace  VariableName=mc_spd_out_a  SampleTime=-1  SaveFormat=Array
  wires:
  In1/1 -> To Workspace/1

== system bd_par_auto2/motor/controller <mc>/motor model & interface/mc model/enhancedToWorkspace9 ==
  In1 : Inport  Port=1  LatchInput=off
  To Workspace : ToWorkspace  VariableName=mc_trq_out_a  SampleTime=-1  SaveFormat=Array
  wires:
  In1/1 -> To Workspace/1

== system bd_par_auto2/motor/controller <mc>/motor model & interface/mc model/mc tmp ==
  Qmc_gen : Inport  Port=1  LatchInput=off
  veh spd : Inport  Port=2  LatchInput=off
  key ON? : Inport  Port=3  LatchInput=off
  Enable : EnablePort  StatesWhenEnabling=reset
  1/mcp : Gain  Gain=1/(mc_mass*mc_cp)  Multiplication=Element-wise(K.*u)  SaturateOnIntegerOverflow=on
  >=0 : Saturate  UpperLimit=Inf  LowerLimit=0  LinearizeAsGain=on
  ">=0 " : Saturate  UpperLimit=Inf  LowerLimit=0  LinearizeAsGain=on
  Block NOTES : Subsystem
      settings: RTWFcnNameOpts=Auto  RTWFileNameOpts=Auto
      mask Display: disp('Block\nNOTES')
  Mux10 : Mux  Inputs=2
      settings: DisplayOption=none
  Mux9 : Mux  Inputs=2
      settings: DisplayOption=none
  Qa : Fcn  Expr=u(1)*(mc_sarea*mc_trq_scale*mc_spd_scale)*u(2)
  Qc1 : Sum  Inputs=-+  SaturateOnIntegerOverflow=on
  Qnet : Sum  Inputs=+++  SaturateOnIntegerOverflow=on
  Qp2a,v7 : Fcn  Expr=amb_tmp-u(1)
  Qr : Fcn  Expr=0.9*(5.67e-8)*(mc_sarea*mc_trq_scale*mc_spd_scale)*((amb_tmp+273)^4 - (u(1)+273)^4)
  Tmc3 : Integrator  ExternalReset=none  InitialConditionSource=internal  InitialCondition=mc_init_tmp  LimitOutput=off  UpperSaturationLimit=inf  LowerSaturationLimit=-inf  ShowSaturationPort=off  ShowStatePort=off  AbsoluteTolerance=auto
  Va/Vv : Gain  Gain=0.5  Multiplication=Element-wise(K.*u)  SaturateOnIntegerOverflow=on
  ha : Fcn  Expr=6 + 6*((abs(u(2))/1000))^0.25 + 60*(abs(u(1))/30)^0.63
  mc coolant : Subsystem  TreatAsAtomicUnit=on
      settings: RTWFcnNameOpts=Auto  RTWFileNameOpts=Auto
  Tmc : Outport  Port=1  InitialOutput=0
  Qmc_clt : Outport  Port=2  OutputWhenDisabled=reset  InitialOutput=0
  wires:
  Qnet/1 -> Qc1/2, mc coolant/2("Qmc ")
  Qc1/1 -> 1/mcp/1
  1/mcp/1 -> Tmc3/1
  Tmc3/1 -> Qp2a,v7/1, Qr/1, Tmc/1, mc coolant/1(Tcl)
  mc coolant/1(Qmc_clt) -> Qc1/1, >=0/1
  >=0/1 -> Qmc_clt/1
  key ON?/1 -> mc coolant/Enable
  veh spd/1 -> Va/Vv/1
  Qa/1 -> Qnet/2
  ">=0 "/1 -> Qnet/1
  Qmc_gen/1 -> ">=0 "/1
  Qr/1 -> Qnet/3
  Qp2a,v7/1 -> Mux10/2, Mux9/2
  ha/1 -> Mux10/1
  Va/Vv/1 -> Mux9/1
  Mux9/1 -> ha/1
  Mux10/1 -> Qa/1

== system bd_par_auto2/motor/controller <mc>/motor model & interface/mc model/motor controller logic interface ==
  w_mc_out_r : Inport  Port=1  LatchInput=off
  P_mc_in_1lim : Inport  Port=2  LatchInput=off
  motor controller logic : Subsystem
      settings: RTWFcnNameOpts=Auto  RTWFileNameOpts=Auto
  P_mc_in_r : Outport  Port=1  InitialOutput=0
  tag scope: P_mc_in_1lim=scoped, P_mc_in_r=scoped, w_mc_out_r=scoped
  wires:
  w_mc_out_r/1 -> [w_mc_out_r], motor controller logic/3(req'd output spd (rad/s))
  P_mc_in_1lim/1 -> [P_mc_in_1lim], motor controller logic/2(req'd input power (W))
  motor controller logic/1(req'd input power (W)1) -> P_mc_in_r/1, [P_mc_in_r]
  [bus_voltage_prev] -> motor controller logic/1(bus voltage  previous)
  [shifting] -> motor controller logic/4(shifting)
